simulink model "ssc_aircraft_ecs_data"  (Simulink 9.1)
settings: Solver=VariableStepAuto  StartTime=0.0  StopTime=6000  RelTol=1e-3  AbsTol=1e-3
PreLoadFcn:
  | p_init = 101.325; % kPa
  | T_init = 45; % degC
  | RH_init = 0.5;
  | O3_init = 0.05e-6;
  | 
  | R_O3 = 173.218; % J/(kg*K)
  | 
  | flow_area = 0.016; % m^2
  | 
  | D_fuselage = 4; % m
  | L_fuselage = 35; % m
undefined symbols (not defined in the file or in its folder): sigbuilder_block
libraries: fl_lib x57, nesl_utility x24, simulink x6, HVAC_lib x4
(part 2 of 2)

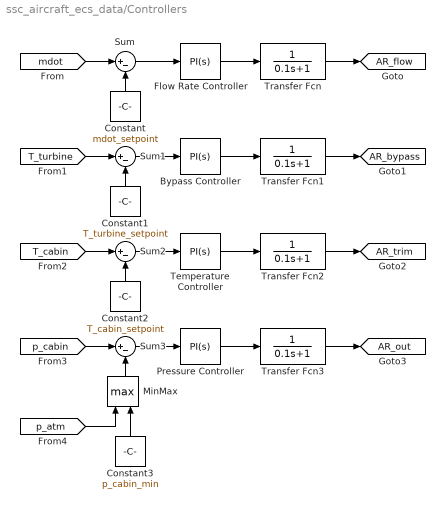
== system ssc_aircraft_ecs_data/Controllers ==
  Bypass Controller : simulink/Continuous/PID Controller  Controller=PI  TimeDomain=Continuous-time  SampleTime=-1  IntegratorMethod=Forward Euler  FilterMethod=Forward Euler  Form=Parallel  UseFilter=on  ControllerParametersSource=internal  P=-flow_area/100  I=-flow_area/100  D=0  N=100  InitialConditionSource=internal  InitialConditionForIntegrator=0  InitialConditionForFilter=0  ExternalReset=none  LimitOutput=on  UpperSaturationLimit=0.95*flow_area  LowerSaturationLimit=1e-9  LinearizeAsGain=on  AntiWindupMode=back-calculation  Kb=1  TrackingMode=off  Kt=1  PParamMin=[]  PParamMax=[]  IParamMin=[]  IParamMax=[]  DParamMin=[]  DParamMax=[]  NParamMin=[]  NParamMax=[]  KbParamMin=[]  KbParamMax=[]  KtParamMin=[]  KtParamMax=[]  POutMin=[]  POutMax=[]  IOutMin=[]  IOutMax=[]  DOutMin=[]  DOutMax=[]  NOutMin=[]  NOutMax=[]  KbOutMin=[]  KbOutMax=[]  KtOutMin=[]  KtOutMax=[]  IntegratorOutMin=[]  IntegratorOutMax=[]  FilterOutMin=[]  FilterOutMax=[]  SumOutMin=[]  SumOutMax=[]  SumI1OutMin=[]  SumI1OutMax=[]  SumI2OutMin=[]  SumI2OutMax=[]  SumI3OutMin=[]  SumI3OutMax=[]  SumDOutMin=[]  SumDOutMax=[]  SaturationOutMin=[]  SaturationOutMax=[]  IntegratorContinuousStateAttributes=''  IntegratorStateMustResolveToSignalObject=off  IntegratorRTWStateStorageClass=Auto  FilterContinuousStateAttributes=''  FilterStateMustResolveToSignalObject=off  FilterRTWStateStorageClass=Auto  DifferentiatorICPrevScaledInput=0  DifferentiatorOutMin=[]  DifferentiatorOutMax=[]  InitialConditionSetting=State (most efficient)  FilterDiffOutCoefMin=[]  FilterDiffOutCoefMax=[]  SumDenOutMin=[]  SumDenOutMax=[]  SumNumOutMin=[]  SumNumOutMax=[]  ReciprocalOutMin=[]  ReciprocalOutMax=[]  DivideOutMin=[]  DivideOutMax=[]  TunerSelectOption=Transfer Function Based (PID Tuner App)
  Constant : Constant  Value=mdot_setpoint
  Constant1 : Constant  Value=T_turbine_setpoint
  Constant2 : Constant  Value=T_cabin_setpoint
  Constant3 : Constant  Value=p_cabin_min
  Flow Rate Controller : simulink/Continuous/PID Controller  Controller=PI  TimeDomain=Continuous-time  SampleTime=-1  IntegratorMethod=Forward Euler  FilterMethod=Forward Euler  Form=Parallel  UseFilter=on  ControllerParametersSource=internal  P=-flow_area/10  I=-flow_area/10  D=0  N=100  InitialConditionSource=internal  InitialConditionForIntegrator=0  InitialConditionForFilter=0  ExternalReset=none  LimitOutput=on  UpperSaturationLimit=0.95*flow_area  LowerSaturationLimit=1e-9  LinearizeAsGain=on  AntiWindupMode=back-calculation  Kb=1  TrackingMode=off  Kt=1  PParamMin=[]  PParamMax=[]  IParamMin=[]  IParamMax=[]  DParamMin=[]  DParamMax=[]  NParamMin=[]  NParamMax=[]  KbParamMin=[]  KbParamMax=[]  KtParamMin=[]  KtParamMax=[]  POutMin=[]  POutMax=[]  IOutMin=[]  IOutMax=[]  DOutMin=[]  DOutMax=[]  NOutMin=[]  NOutMax=[]  KbOutMin=[]  KbOutMax=[]  KtOutMin=[]  KtOutMax=[]  IntegratorOutMin=[]  IntegratorOutMax=[]  FilterOutMin=[]  FilterOutMax=[]  SumOutMin=[]  SumOutMax=[]  SumI1OutMin=[]  SumI1OutMax=[]  SumI2OutMin=[]  SumI2OutMax=[]  SumI3OutMin=[]  SumI3OutMax=[]  SumDOutMin=[]  SumDOutMax=[]  SaturationOutMin=[]  SaturationOutMax=[]  IntegratorContinuousStateAttributes=''  IntegratorStateMustResolveToSignalObject=off  IntegratorRTWStateStorageClass=Auto  FilterContinuousStateAttributes=''  FilterStateMustResolveToSignalObject=off  FilterRTWStateStorageClass=Auto  DifferentiatorICPrevScaledInput=0  DifferentiatorOutMin=[]  DifferentiatorOutMax=[]  InitialConditionSetting=State (most efficient)  FilterDiffOutCoefMin=[]  FilterDiffOutCoefMax=[]  SumDenOutMin=[]  SumDenOutMax=[]  SumNumOutMin=[]  SumNumOutMax=[]  ReciprocalOutMin=[]  ReciprocalOutMax=[]  DivideOutMin=[]  DivideOutMax=[]  TunerSelectOption=Transfer Function Based (PID Tuner App)
  MinMax : MinMax  Function=max  Inputs=2
  Pressure Controller : simulink/Continuous/PID Controller  Controller=PI  TimeDomain=Continuous-time  SampleTime=-1  IntegratorMethod=Forward Euler  FilterMethod=Forward Euler  Form=Parallel  UseFilter=on  ControllerParametersSource=internal  P=flow_area/100  I=flow_area/100  D=0  N=100  InitialConditionSource=internal  InitialConditionForIntegrator=0  InitialConditionForFilter=0  ExternalReset=none  LimitOutput=on  UpperSaturationLimit=0.95*flow_area  LowerSaturationLimit=1e-9  LinearizeAsGain=on  AntiWindupMode=back-calculation  Kb=1  TrackingMode=off  Kt=1  PParamMin=[]  PParamMax=[]  IParamMin=[]  IParamMax=[]  DParamMin=[]  DParamMax=[]  NParamMin=[]  NParamMax=[]  KbParamMin=[]  KbParamMax=[]  KtParamMin=[]  KtParamMax=[]  POutMin=[]  POutMax=[]  IOutMin=[]  IOutMax=[]  DOutMin=[]  DOutMax=[]  NOutMin=[]  NOutMax=[]  KbOutMin=[]  KbOutMax=[]  KtOutMin=[]  KtOutMax=[]  IntegratorOutMin=[]  IntegratorOutMax=[]  FilterOutMin=[]  FilterOutMax=[]  SumOutMin=[]  SumOutMax=[]  SumI1OutMin=[]  SumI1OutMax=[]  SumI2OutMin=[]  SumI2OutMax=[]  SumI3OutMin=[]  SumI3OutMax=[]  SumDOutMin=[]  SumDOutMax=[]  SaturationOutMin=[]  SaturationOutMax=[]  IntegratorContinuousStateAttributes=''  IntegratorStateMustResolveToSignalObject=off  IntegratorRTWStateStorageClass=Auto  FilterContinuousStateAttributes=''  FilterStateMustResolveToSignalObject=off  FilterRTWStateStorageClass=Auto  DifferentiatorICPrevScaledInput=0  DifferentiatorOutMin=[]  DifferentiatorOutMax=[]  InitialConditionSetting=State (most efficient)  FilterDiffOutCoefMin=[]  FilterDiffOutCoefMax=[]  SumDenOutMin=[]  SumDenOutMax=[]  SumNumOutMin=[]  SumNumOutMax=[]  ReciprocalOutMin=[]  ReciprocalOutMax=[]  DivideOutMin=[]  DivideOutMax=[]  TunerSelectOption=Transfer Function Based (PID Tuner App)
  Sum{,1..3} (4 alike) : Sum  Inputs=|+-
  Temperature Controller : simulink/Continuous/PID Controller  Controller=PI  TimeDomain=Continuous-time  SampleTime=-1  IntegratorMethod=Forward Euler  FilterMethod=Forward Euler  Form=Parallel  UseFilter=on  ControllerParametersSource=internal  P=-flow_area/100  I=-flow_area/100  D=0  N=100  InitialConditionSource=internal  InitialConditionForIntegrator=0  InitialConditionForFilter=0  ExternalReset=none  LimitOutput=on  UpperSaturationLimit=0.95*flow_area  LowerSaturationLimit=1e-9  LinearizeAsGain=on  AntiWindupMode=back-calculation  Kb=1  TrackingMode=off  Kt=1  PParamMin=[]  PParamMax=[]  IParamMin=[]  IParamMax=[]  DParamMin=[]  DParamMax=[]  NParamMin=[]  NParamMax=[]  KbParamMin=[]  KbParamMax=[]  KtParamMin=[]  KtParamMax=[]  POutMin=[]  POutMax=[]  IOutMin=[]  IOutMax=[]  DOutMin=[]  DOutMax=[]  NOutMin=[]  NOutMax=[]  KbOutMin=[]  KbOutMax=[]  KtOutMin=[]  KtOutMax=[]  IntegratorOutMin=[]  IntegratorOutMax=[]  FilterOutMin=[]  FilterOutMax=[]  SumOutMin=[]  SumOutMax=[]  SumI1OutMin=[]  SumI1OutMax=[]  SumI2OutMin=[]  SumI2OutMax=[]  SumI3OutMin=[]  SumI3OutMax=[]  SumDOutMin=[]  SumDOutMax=[]  SaturationOutMin=[]  SaturationOutMax=[]  IntegratorContinuousStateAttributes=''  IntegratorStateMustResolveToSignalObject=off  IntegratorRTWStateStorageClass=Auto  FilterContinuousStateAttributes=''  FilterStateMustResolveToSignalObject=off  FilterRTWStateStorageClass=Auto  DifferentiatorICPrevScaledInput=0  DifferentiatorOutMin=[]  DifferentiatorOutMax=[]  InitialConditionSetting=State (most efficient)  FilterDiffOutCoefMin=[]  FilterDiffOutCoefMax=[]  SumDenOutMin=[]  SumDenOutMax=[]  SumNumOutMin=[]  SumNumOutMax=[]  ReciprocalOutMin=[]  ReciprocalOutMax=[]  DivideOutMin=[]  DivideOutMax=[]  TunerSelectOption=Transfer Function Based (PID Tuner App)
  Transfer Fcn{,1..3} (4 alike) : TransferFcn  Denominator=[0.1 1]
  tag scope: AR_bypass=global, AR_flow=global, AR_out=global, AR_trim=global
  wires:
  Flow Rate Controller/1 -> Transfer Fcn/1
  Sum/1 -> Flow Rate Controller/1
  Constant/1 -> Sum/2
  [mdot] -> Sum/1
  Bypass Controller/1 -> Transfer Fcn1/1
  Temperature Controller/1 -> Transfer Fcn2/1
  Pressure Controller/1 -> Transfer Fcn3/1
  Sum1/1 -> Bypass Controller/1
  [T_turbine] -> Sum1/1
  Sum2/1 -> Temperature Controller/1
  Sum3/1 -> Pressure Controller/1
  [T_cabin] -> Sum2/1
  [p_cabin] -> Sum3/1
  Constant1/1 -> Sum1/2
  Constant2/1 -> Sum2/2
  MinMax/1 -> Sum3/2
  [p_atm] -> MinMax/1
  Constant3/1 -> MinMax/2
  Transfer Fcn/1 -> [AR_flow]
  Transfer Fcn1/1 -> [AR_bypass]
  Transfer Fcn2/1 -> [AR_trim]
  Transfer Fcn3/1 -> [AR_out]

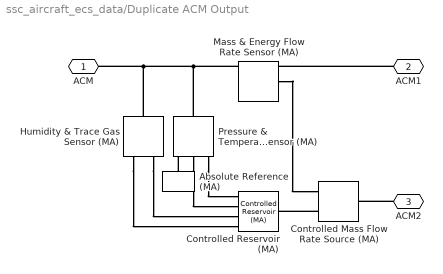
== system ssc_aircraft_ecs_data/Duplicate ACM Output ==
  Absolute Reference (MA) : fl_lib/Moist Air/Elements/Absolute Reference (MA)
      settings: SourceProductName=Simscape  SourceProductBaseCode=SS
  Controlled Mass Flow Rate Source (MA) : fl_lib/Moist Air/Sources/Controlled Mass Flow Rate Source (MA)  power_spec=foundation.enum.power_spec.none  area_A=flow_area m^2  area_B=flow_area m^2
      settings: SourceProductName=Simscape  SourceProductBaseCode=SS
  Controlled Reservoir (MA) : fl_lib/Moist Air/Elements/Controlled Reservoir (MA)  moisture_spec=foundation.enum.moisture_spec.specific_humidity  trace_gas_spec=foundation.enum.trace_gas_spec.mass_fraction  RH_ws=1  area_A=flow_area m^2  input_error_spec=foundation.enum.input_range_error.limit
      settings: SourceProductName=Simscape  SourceProductBaseCode=SS
  Humidity & Trace Gas Sensor (MA) : fl_lib/Moist Air/Sensors/Humidity & Trace Gas Sensor (MA)  moisture_spec=foundation.enum.moisture_spec.specific_humidity  trace_gas_spec=foundation.enum.trace_gas_spec.mass_fraction
      settings: SourceProductName=Simscape  SourceProductBaseCode=SS
  Mass & Energy Flow Rate Sensor (MA) : fl_lib/Moist Air/Sensors/Mass & Energy Flow Rate Sensor (MA)
      settings: SourceProductName=Simscape  SourceProductBaseCode=SS
  Pressure & Temperature Sensor (MA) : fl_lib/Moist Air/Sensors/Pressure & Temperature Sensor (MA)
      settings: SourceProductName=Simscape  SourceProductBaseCode=SS
  ACM : PMIOPort  Side=Left
  ACM1 : PMIOPort  Port=2  Side=Right
  ACM2 : PMIOPort  Port=3  Side=Right
  connections:
  ACM1/RConn1 -- Mass & Energy Flow Rate Sensor (MA)/RConn1
  Mass & Energy Flow Rate Sensor (MA)/LConn1 -- ACM/RConn1 -- Humidity & Trace Gas Sensor (MA)/LConn1 -- Pressure & Temperature Sensor (MA)/LConn1
  Controlled Mass Flow Rate Source (MA)/LConn1 -- Controlled Reservoir (MA)/LConn1
  ACM2/RConn1 -- Controlled Mass Flow Rate Source (MA)/RConn1
  Mass & Energy Flow Rate Sensor (MA)/RConn2 -- Controlled Mass Flow Rate Source (MA)/LConn2
  Humidity & Trace Gas Sensor (MA)/RConn1 -- Controlled Reservoir (MA)/RConn3
  Humidity & Trace Gas Sensor (MA)/RConn2 -- Controlled Reservoir (MA)/RConn4
  Absolute Reference (MA)/LConn1 -- Pressure & Temperature Sensor (MA)/RConn1
  Pressure & Temperature Sensor (MA)/RConn3 -- Controlled Reservoir (MA)/RConn1
  Pressure & Temperature Sensor (MA)/RConn2 -- Controlled Reservoir (MA)/RConn2

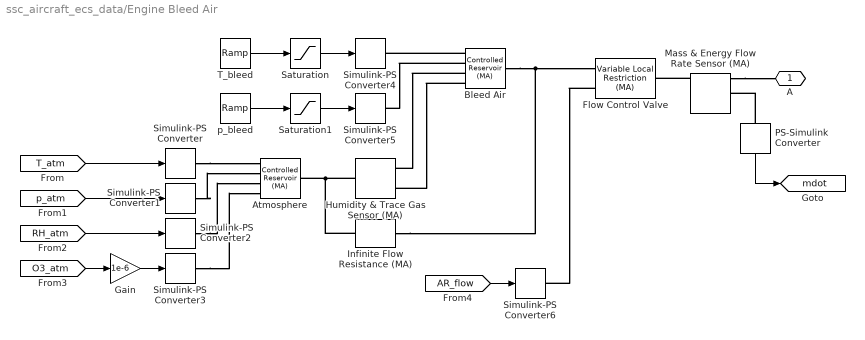
== system ssc_aircraft_ecs_data/Engine Bleed Air ==
  Atmosphere : fl_lib/Moist Air/Elements/Controlled Reservoir (MA)  moisture_spec=foundation.enum.moisture_spec.relative_humidity  trace_gas_spec=foundation.enum.trace_gas_spec.mole_fraction  RH_ws=1  area_A=flow_area m^2  input_error_spec=foundation.enum.input_range_error.warn
      settings: SourceProductName=Simscape  SourceProductBaseCode=SS
  Bleed Air : fl_lib/Moist Air/Elements/Controlled Reservoir (MA)  moisture_spec=foundation.enum.moisture_spec.specific_humidity  trace_gas_spec=foundation.enum.trace_gas_spec.mass_fraction  RH_ws=1  area_A=flow_area m^2  input_error_spec=foundation.enum.input_range_error.warn
      settings: SourceProductName=Simscape  SourceProductBaseCode=SS
  Flow Control Valve : fl_lib/Moist Air/Elements/Variable Local Restriction (MA)  min_area=1e-10 m^2  max_area=0.98*flow_area m^2  area=flow_area m^2  Cd=0.8  B_lam=0.999
      settings: SourceProductName=Simscape  SourceProductBaseCode=SS
  Gain : Gain  Gain=1e-6
  Humidity & Trace Gas Sensor (MA) : fl_lib/Moist Air/Sensors/Humidity & Trace Gas Sensor (MA)  moisture_spec=foundation.enum.moisture_spec.specific_humidity  trace_gas_spec=foundation.enum.trace_gas_spec.mass_fraction
      settings: SourceProductName=Simscape  SourceProductBaseCode=SS
  Infinite Flow Resistance (MA) : fl_lib/Moist Air/Elements/Infinite Flow Resistance (MA)  p_specify=off  p_priority=None  p=0 MPa  p_nominal_specify=off  p_nominal_unit=MPa  p_nominal_value=1  T_specify=off  T_priority=None  T=0 K  T_nominal_specify=off  T_nominal_unit=K  T_nominal_value=1  x_w_specify=off  x_w_priority=None  x_w=0  x_w_nominal_specify=off  x_w_nominal_unit=1  x_w_nominal_value=1  x_g_specify=off  x_g_priority=None  x_g=0  x_g_nominal_specify=off  x_g_nominal_unit=1  x_g_nominal_value=1
      settings: SourceProductName=Simscape  SourceProductBaseCode=SS
  Mass & Energy Flow Rate Sensor (MA) : fl_lib/Moist Air/Sensors/Mass & Energy Flow Rate Sensor (MA)
      settings: SourceProductName=Simscape  SourceProductBaseCode=SS
  PS-Simulink Converter : nesl_utility/PS-Simulink Converter  PhysicalDomain=network_engine_domain  SubClassName=ps_output  LeftPortType=input  RightPortType=output  PseudoPeriodic=off  Frequencies=[]  Unit=kg/s  AffineConversion=off
  Saturation : Saturate  UpperLimit=T_bleed  LowerLimit=-inf
  Saturation1 : Saturate  UpperLimit=p_bleed  LowerLimit=-inf
  Simulink-PS Converter : nesl_utility/Simulink-PS Converter  PhysicalDomain=network_engine_domain  SubClassName=ps_input  LeftPortType=input  RightPortType=output  PseudoPeriodic=off  Frequencies=[]  NoiseDistribution=none  NoiseParameters=[]  Unit=degC  AffineConversion=on  FilteringAndDerivatives=provide  SimscapeFilterOrder=1  InputFilterTimeConstant=0.001  UdotUserProvided=0
  Simulink-PS Converter1 : nesl_utility/Simulink-PS Converter  PhysicalDomain=network_engine_domain  SubClassName=ps_input  LeftPortType=input  RightPortType=output  PseudoPeriodic=off  Frequencies=[]  NoiseDistribution=none  NoiseParameters=[]  Unit=kPa  AffineConversion=off  FilteringAndDerivatives=provide  SimscapeFilterOrder=1  InputFilterTimeConstant=0.001  UdotUserProvided=0
  Simulink-PS Converter2 : nesl_utility/Simulink-PS Converter  PhysicalDomain=network_engine_domain  SubClassName=ps_input  LeftPortType=input  RightPortType=output  PseudoPeriodic=off  Frequencies=[]  NoiseDistribution=none  NoiseParameters=[]  Unit=1  AffineConversion=off  FilteringAndDerivatives=provide  SimscapeFilterOrder=1  InputFilterTimeConstant=0.001  UdotUserProvided=0
  Simulink-PS Converter3 : nesl_utility/Simulink-PS Converter  PhysicalDomain=network_engine_domain  SubClassName=ps_input  LeftPortType=input  RightPortType=output  PseudoPeriodic=off  Frequencies=[]  NoiseDistribution=none  NoiseParameters=[]  Unit=1  AffineConversion=off  FilteringAndDerivatives=provide  SimscapeFilterOrder=1  InputFilterTimeConstant=0.001  UdotUserProvided=0
  Simulink-PS Converter4 : nesl_utility/Simulink-PS Converter  PhysicalDomain=network_engine_domain  SubClassName=ps_input  LeftPortType=input  RightPortType=output  PseudoPeriodic=off  Frequencies=[]  NoiseDistribution=none  NoiseParameters=[]  Unit=degC  AffineConversion=on  FilteringAndDerivatives=provide  SimscapeFilterOrder=1  InputFilterTimeConstant=0.001  UdotUserProvided=0
  Simulink-PS Converter5 : nesl_utility/Simulink-PS Converter  PhysicalDomain=network_engine_domain  SubClassName=ps_input  LeftPortType=input  RightPortType=output  PseudoPeriodic=off  Frequencies=[]  NoiseDistribution=none  NoiseParameters=[]  Unit=kPa  AffineConversion=off  FilteringAndDerivatives=provide  SimscapeFilterOrder=1  InputFilterTimeConstant=0.001  UdotUserProvided=0
  Simulink-PS Converter6 : nesl_utility/Simulink-PS Converter  PhysicalDomain=network_engine_domain  SubClassName=ps_input  LeftPortType=input  RightPortType=output  PseudoPeriodic=off  Frequencies=[]  NoiseDistribution=none  NoiseParameters=[]  Unit=m^2  AffineConversion=off  FilteringAndDerivatives=provide  SimscapeFilterOrder=1  InputFilterTimeConstant=0.001  UdotUserProvided=0
  T_bleed : simulink/Sources/Ramp  slope=(T_bleed - T_init)/10  start=0  InitialOutput=T_init
  p_bleed : simulink/Sources/Ramp  slope=(p_bleed - p_init)/10  start=0  InitialOutput=p_init
  A : PMIOPort  Side=Right
  tag scope: mdot=global
  wires:
  Saturation/1 -> Simulink-PS Converter4/1
  Saturation1/1 -> Simulink-PS Converter5/1
  [T_atm] -> Simulink-PS Converter/1
  [p_atm] -> Simulink-PS Converter1/1
  [RH_atm] -> Simulink-PS Converter2/1
  [O3_atm] -> Gain/1
  [AR_flow] -> Simulink-PS Converter6/1
  PS-Simulink Converter/1 -> [mdot]
  Gain/1 -> Simulink-PS Converter3/1
  T_bleed/1 -> Saturation/1
  p_bleed/1 -> Saturation1/1
  connections:
  Flow Control Valve/LConn2 -- Simulink-PS Converter6/RConn1
  Bleed Air/LConn1 -- Infinite Flow Resistance (MA)/RConn1 -- Flow Control Valve/LConn1
  Bleed Air/RConn2 -- Simulink-PS Converter5/RConn1
  Bleed Air/RConn1 -- Simulink-PS Converter4/RConn1
  Bleed Air/RConn4 -- Humidity & Trace Gas Sensor (MA)/RConn2
  Bleed Air/RConn3 -- Humidity & Trace Gas Sensor (MA)/RConn1
  PS-Simulink Converter/LConn1 -- Mass & Energy Flow Rate Sensor (MA)/RConn2
  Humidity & Trace Gas Sensor (MA)/LConn1 -- Infinite Flow Resistance (MA)/LConn1 -- Atmosphere/LConn1
  Simulink-PS Converter/RConn1 -- Atmosphere/RConn1
  Simulink-PS Converter1/RConn1 -- Atmosphere/RConn2
  Simulink-PS Converter2/RConn1 -- Atmosphere/RConn3
  Simulink-PS Converter3/RConn1 -- Atmosphere/RConn4
  Mass & Energy Flow Rate Sensor (MA)/RConn1 -- A/RConn1
  Mass & Energy Flow Rate Sensor (MA)/LConn1 -- Flow Control Valve/RConn1

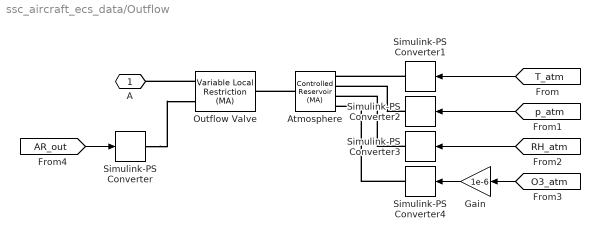
== system ssc_aircraft_ecs_data/Outflow ==
  Atmosphere : fl_lib/Moist Air/Elements/Controlled Reservoir (MA)  moisture_spec=foundation.enum.moisture_spec.relative_humidity  trace_gas_spec=foundation.enum.trace_gas_spec.mole_fraction  RH_ws=1  area_A=flow_area m^2  input_error_spec=foundation.enum.input_range_error.warn
      settings: SourceProductName=Simscape  SourceProductBaseCode=SS
  Gain : Gain  Gain=1e-6
  Outflow Valve : fl_lib/Moist Air/Elements/Variable Local Restriction (MA)  min_area=1e-10 m^2  max_area=0.98*flow_area m^2  area=flow_area m^2  Cd=0.8  B_lam=0.999
      settings: SourceProductName=Simscape  SourceProductBaseCode=SS
  Simulink-PS Converter : nesl_utility/Simulink-PS Converter  PhysicalDomain=network_engine_domain  SubClassName=ps_input  LeftPortType=input  RightPortType=output  PseudoPeriodic=off  Frequencies=[]  NoiseDistribution=none  NoiseParameters=[]  Unit=m^2  AffineConversion=off  FilteringAndDerivatives=provide  SimscapeFilterOrder=1  InputFilterTimeConstant=0.001  UdotUserProvided=0
  Simulink-PS Converter1 : nesl_utility/Simulink-PS Converter  PhysicalDomain=network_engine_domain  SubClassName=ps_input  LeftPortType=input  RightPortType=output  PseudoPeriodic=off  Frequencies=[]  NoiseDistribution=none  NoiseParameters=[]  Unit=degC  AffineConversion=on  FilteringAndDerivatives=provide  SimscapeFilterOrder=1  InputFilterTimeConstant=0.001  UdotUserProvided=0
  Simulink-PS Converter2 : nesl_utility/Simulink-PS Converter  PhysicalDomain=network_engine_domain  SubClassName=ps_input  LeftPortType=input  RightPortType=output  PseudoPeriodic=off  Frequencies=[]  NoiseDistribution=none  NoiseParameters=[]  Unit=kPa  AffineConversion=off  FilteringAndDerivatives=provide  SimscapeFilterOrder=1  InputFilterTimeConstant=0.001  UdotUserProvided=0
  Simulink-PS Converter3 : nesl_utility/Simulink-PS Converter  PhysicalDomain=network_engine_domain  SubClassName=ps_input  LeftPortType=input  RightPortType=output  PseudoPeriodic=off  Frequencies=[]  NoiseDistribution=none  NoiseParameters=[]  Unit=1  AffineConversion=off  FilteringAndDerivatives=provide  SimscapeFilterOrder=1  InputFilterTimeConstant=0.001  UdotUserProvided=0
  Simulink-PS Converter4 : nesl_utility/Simulink-PS Converter  PhysicalDomain=network_engine_domain  SubClassName=ps_input  LeftPortType=input  RightPortType=output  PseudoPeriodic=off  Frequencies=[]  NoiseDistribution=none  NoiseParameters=[]  Unit=1  AffineConversion=off  FilteringAndDerivatives=provide  SimscapeFilterOrder=1  InputFilterTimeConstant=0.001  UdotUserProvided=0
  A : PMIOPort  Side=Left
  wires:
  [T_atm] -> Simulink-PS Converter1/1
  [p_atm] -> Simulink-PS Converter2/1
  [RH_atm] -> Simulink-PS Converter3/1
  [O3_atm] -> Gain/1
  [AR_out] -> Simulink-PS Converter/1
  Gain/1 -> Simulink-PS Converter4/1
  connections:
  Atmosphere/LConn1 -- Outflow Valve/RConn1
  Outflow Valve/LConn1 -- A/RConn1
  Simulink-PS Converter2/RConn1 -- Atmosphere/RConn2
  Simulink-PS Converter1/RConn1 -- Atmosphere/RConn1
  Simulink-PS Converter3/RConn1 -- Atmosphere/RConn3
  Simulink-PS Converter4/RConn1 -- Atmosphere/RConn4
  Simulink-PS Converter/RConn1 -- Outflow Valve/LConn2

== system ssc_aircraft_ecs_data/Ram Air ==
  Constant : Constant  Value=mdot_ram
  Simulink-PS Converter : nesl_utility/Simulink-PS Converter  PhysicalDomain=network_engine_domain  SubClassName=ps_input  LeftPortType=input  RightPortType=output  PseudoPeriodic=off  Frequencies=[]  NoiseDistribution=none  NoiseParameters=[]  Unit=degC  AffineConversion=on  FilteringAndDerivatives=provide  SimscapeFilterOrder=1  InputFilterTimeConstant=0.001  UdotUserProvided=0
  Simulink-PS Converter1 : nesl_utility/Simulink-PS Converter  PhysicalDomain=network_engine_domain  SubClassName=ps_input  LeftPortType=input  RightPortType=output  PseudoPeriodic=off  Frequencies=[]  NoiseDistribution=none  NoiseParameters=[]  Unit=kg/s  AffineConversion=off  FilteringAndDerivatives=provide  SimscapeFilterOrder=1  InputFilterTimeConstant=0.001  UdotUserProvided=0
  T : PMIOPort  Side=Right
  M : PMIOPort  Port=2  Side=Right
  wires:
  [T_rec] -> Simulink-PS Converter/1
  Constant/1 -> Simulink-PS Converter1/1
  connections:
  Simulink-PS Converter/RConn1 -- T/RConn1
  Simulink-PS Converter1/RConn1 -- M/RConn1

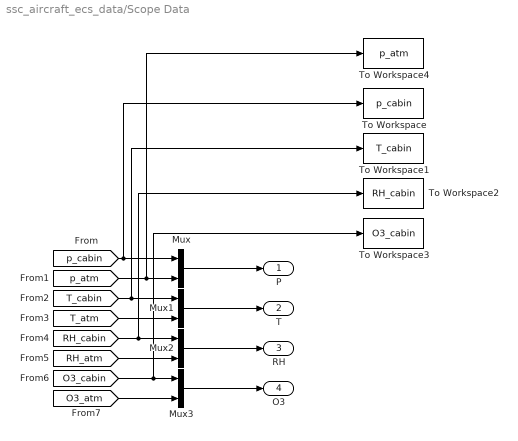
== system ssc_aircraft_ecs_data/Scope Data ==
  Mux{,1..3} (4 alike) : Mux  Inputs=2
  To Workspace : ToWorkspace  VariableName=p_cabin  SampleTime=1
  To Workspace1 : ToWorkspace  VariableName=T_cabin  SampleTime=1
  To Workspace2 : ToWorkspace  VariableName=RH_cabin  SampleTime=1
  To Workspace3 : ToWorkspace  VariableName=O3_cabin  SampleTime=1
  To Workspace4 : ToWorkspace  VariableName=p_atm  SampleTime=1
  P : Outport
  T : Outport  Port=2
  RH : Outport  Port=3
  O3 : Outport  Port=4
  wires:
  [p_cabin] -> To Workspace/1, Mux/1
  [T_atm] -> Mux1/2
  [p_atm] -> To Workspace4/1, Mux/2
  [RH_atm] -> Mux2/2
  [T_cabin] -> To Workspace1/1, Mux1/1
  [O3_cabin] -> To Workspace3/1, Mux3/1
  [RH_cabin] -> To Workspace2/1, Mux2/1
  [O3_atm] -> Mux3/2
  Mux2/1 -> RH/1
  Mux/1 -> P/1
  Mux1/1 -> T/1
  Mux3/1 -> O3/1

== system ssc_aircraft_ecs_data/T,s 1 ==
  Thermodynamic Properties Sensor (MA) : fl_lib/Moist Air/Sensors/Thermodynamic Properties Sensor (MA)
      settings: SourceProductName=Simscape  SourceProductBaseCode=SS
  A : PMIOPort  Side=Left
  connections:
  Thermodynamic Properties Sensor (MA)/LConn1 -- A/RConn1

== system ssc_aircraft_ecs_data/T,s 2 ==
  Thermodynamic Properties Sensor (MA) : fl_lib/Moist Air/Sensors/Thermodynamic Properties Sensor (MA)
      settings: SourceProductName=Simscape  SourceProductBaseCode=SS
  A : PMIOPort  Side=Left
  connections:
  Thermodynamic Properties Sensor (MA)/LConn1 -- A/RConn1

== system ssc_aircraft_ecs_data/T,s 3 ==
  Thermodynamic Properties Sensor (MA) : fl_lib/Moist Air/Sensors/Thermodynamic Properties Sensor (MA)
      settings: SourceProductName=Simscape  SourceProductBaseCode=SS
  A : PMIOPort  Side=Left
  connections:
  Thermodynamic Properties Sensor (MA)/LConn1 -- A/RConn1

== system ssc_aircraft_ecs_data/T,s 4 ==
  Thermodynamic Properties Sensor (MA) : fl_lib/Moist Air/Sensors/Thermodynamic Properties Sensor (MA)
      settings: SourceProductName=Simscape  SourceProductBaseCode=SS
  A : PMIOPort  Side=Left
  connections:
  Thermodynamic Properties Sensor (MA)/LConn1 -- A/RConn1

== system ssc_aircraft_ecs_data/T,s 5 ==
  Absolute Reference (MA) : fl_lib/Moist Air/Elements/Absolute Reference (MA)
      settings: SourceProductName=Simscape  SourceProductBaseCode=SS
  PS-Simulink Converter : nesl_utility/PS-Simulink Converter  PhysicalDomain=network_engine_domain  SubClassName=ps_output  LeftPortType=input  RightPortType=output  PseudoPeriodic=off  Frequencies=[]  Unit=degC  AffineConversion=on
  Pressure & Temperature Sensor (MA) : fl_lib/Moist Air/Sensors/Pressure & Temperature Sensor (MA)
      settings: SourceProductName=Simscape  SourceProductBaseCode=SS
  Thermodynamic Properties Sensor (MA) : fl_lib/Moist Air/Sensors/Thermodynamic Properties Sensor (MA)
      settings: SourceProductName=Simscape  SourceProductBaseCode=SS
  A : PMIOPort  Side=Left
  tag scope: T_turbine=global
  wires:
  PS-Simulink Converter/1 -> [T_turbine]
  connections:
  Thermodynamic Properties Sensor (MA)/LConn1 -- A/RConn1 -- Pressure & Temperature Sensor (MA)/LConn1
  Pressure & Temperature Sensor (MA)/RConn3 -- PS-Simulink Converter/LConn1
  Absolute Reference (MA)/LConn1 -- Pressure & Temperature Sensor (MA)/RConn1

== system ssc_aircraft_ecs_data/T,s 6 ==
  Thermodynamic Properties Sensor (MA) : fl_lib/Moist Air/Sensors/Thermodynamic Properties Sensor (MA)
      settings: SourceProductName=Simscape  SourceProductBaseCode=SS
  A : PMIOPort  Side=Left
  connections:
  Thermodynamic Properties Sensor (MA)/LConn1 -- A/RConn1

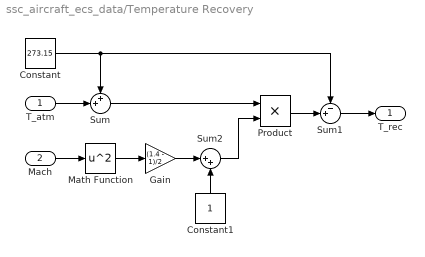
== system ssc_aircraft_ecs_data/Temperature Recovery ==
  T_atm : Inport
  Mach : Inport  Port=2
  Constant : Constant  Value=273.15
  Constant1 : Constant
  Gain : Gain  Gain=(1.4 - 1)/2
  Math Function : Math  Operator=square  SaturateOnIntegerOverflow=on
  Product : Product
  Sum : Sum  Inputs=++|
  Sum1 : Sum  Inputs=-+|
  Sum2 : Sum  Inputs=|++
  T_rec : Outport
  wires:
  T_atm/1 -> Sum/2
  Sum1/1 -> T_rec/1
  Constant/1 -> Sum1/1, Sum/1
  Mach/1 -> Math Function/1
  Math Function/1 -> Gain/1
  Gain/1 -> Sum2/1
  Constant1/1 -> Sum2/2
  Product/1 -> Sum1/2
  Sum2/1 -> Product/2
  Sum/1 -> Product/1

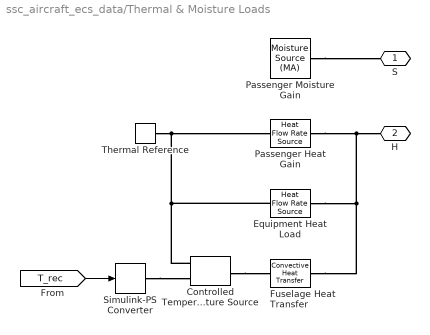
== system ssc_aircraft_ecs_data/Thermal & Moisture Loads ==
  Controlled Temperature Source : fl_lib/Thermal/Thermal Sources/Controlled Temperature Source
      settings: SourceProductName=Simscape
  Equipment Heat Load : fl_lib/Thermal/Thermal Sources/Heat Flow Rate Source  heat_flow=Q_equipment W
      settings: SourceProductName=Simscape  SourceProductBaseCode=SS
  Fuselage Heat Transfer : fl_lib/Thermal/Thermal Elements/Convective Heat Transfer  area=pi * D_fuselage * L_fuselage m^2  heat_tr_coeff=hc_fuselage W/(m^2 * K)  T_specify=off  T_priority=None  T=0 K  T_nominal_specify=off  T_nominal_unit=K  T_nominal_value=1  Q_specify=off  Q_priority=None  Q=0 W  Q_nominal_specify=off  Q_nominal_unit=W  Q_nominal_value=1
  Passenger Heat Gain : fl_lib/Thermal/Thermal Sources/Heat Flow Rate Source  heat_flow=Q_passenger * N_passenger W
      settings: SourceProductName=Simscape  SourceProductBaseCode=SS
  Passenger Moisture Gain : fl_lib/Moist Air/Sources/Moisture & Trace Gas Sources/Moisture Source (MA)  moisture_source_spec=foundation.enum.moisture_source_spec.vapor  moisture_mass_flow=W_passenger * N_passenger g/s  temperature_spec=2  moisture_temperature=T_passenger degC
      settings: SourceProductName=Simscape  SourceProductBaseCode=SS
  Simulink-PS Converter : nesl_utility/Simulink-PS Converter  PhysicalDomain=network_engine_domain  SubClassName=ps_input  LeftPortType=input  RightPortType=output  PseudoPeriodic=off  Frequencies=[]  NoiseDistribution=none  NoiseParameters=[]  Unit=degC  AffineConversion=on  FilteringAndDerivatives=provide  SimscapeFilterOrder=1  InputFilterTimeConstant=0.001  UdotUserProvided=0
  Thermal Reference : fl_lib/Thermal/Thermal Elements/Thermal Reference
  S : PMIOPort  Side=Right
  H : PMIOPort  Port=2  Side=Right
  wires:
  [T_rec] -> Simulink-PS Converter/1
  connections:
  Passenger Moisture Gain/LConn1 -- S/RConn1
  Passenger Heat Gain/LConn1 -- Equipment Heat Load/LConn1 -- Fuselage Heat Transfer/RConn1 -- H/RConn1
  Controlled Temperature Source/LConn1 -- Fuselage Heat Transfer/LConn1
  Thermal Reference/LConn1 -- Equipment Heat Load/RConn1 -- Controlled Temperature Source/RConn2 -- Passenger Heat Gain/RConn1
  Simulink-PS Converter/RConn1 -- Controlled Temperature Source/RConn1

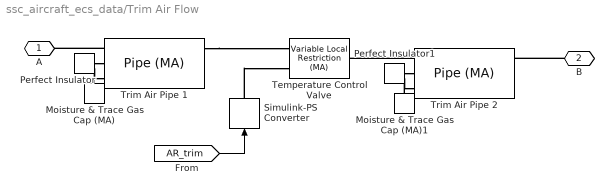
== system ssc_aircraft_ecs_data/Trim Air Flow ==
  Moisture & Trace Gas Cap (MA) : fl_lib/Moist Air/Sources/Moisture & Trace Gas Sources/Moisture & Trace Gas Cap (MA)
      settings: SourceProductName=Simscape  SourceProductBaseCode=SS
  Moisture & Trace Gas Cap (MA)1 : fl_lib/Moist Air/Sources/Moisture & Trace Gas Sources/Moisture & Trace Gas Cap (MA)
      settings: SourceProductName=Simscape  SourceProductBaseCode=SS
  Perfect Insulator : fl_lib/Thermal/Thermal Elements/Perfect Insulator  T_specify=off  T_priority=None  T=0 K  T_nominal_specify=off  T_nominal_unit=K  T_nominal_value=1
      settings: SourceProductName=Simscape
  Perfect Insulator1 : fl_lib/Thermal/Thermal Elements/Perfect Insulator  T_specify=off  T_priority=None  T=0 K  T_nominal_specify=off  T_nominal_unit=K  T_nominal_value=1
      settings: SourceProductName=Simscape
  Simulink-PS Converter : nesl_utility/Simulink-PS Converter  PhysicalDomain=network_engine_domain  SubClassName=ps_input  LeftPortType=input  RightPortType=output  PseudoPeriodic=off  Frequencies=[]  NoiseDistribution=none  NoiseParameters=[]  Unit=m^2  AffineConversion=off  FilteringAndDerivatives=provide  SimscapeFilterOrder=1  InputFilterTimeConstant=0.001  UdotUserProvided=0
  Temperature Control Valve : fl_lib/Moist Air/Elements/Variable Local Restriction (MA)  min_area=1e-10 m^2  max_area=0.98*flow_area m^2  area=flow_area m^2  Cd=0.8  B_lam=0.999
      settings: SourceProductName=Simscape  SourceProductBaseCode=SS
  Trim Air Pipe 1 : fl_lib/Moist Air/Elements/Pipe (MA)  length=1 m  area=flow_area m^2  Dh=sqrt(flow_area*4/pi) m  length_add=0.1 m  roughness=15e-6 m  Re_lam=2000  Re_tur=4000  shape_factor=64  Nu_lam=3.66  RH_ws=1  time_constant=1e-3 s  p_I_specify=on  p_I_priority=High  p_I=p_init kPa  p_I_nominal_specify=off  p_I_nominal_unit=MPa  p_I_nominal_value=1  T_I_specify=on  T_I_priority=High  T_I=T_init degC  T_I_nominal_specify=off  T_I_nominal_unit=K  T_I_nominal_value=1  RH_I_specify=on  RH_I_priority=High  RH_I=RH_init  RH_I_nominal_specify=off  RH_I_nominal_unit=1  RH_I_nominal_value=1  x_w_I_specify=off  x_w_I_priority=None  x_w_I=0  x_w_I_nominal_specify=off  x_w_I_nominal_unit=1  x_w_I_nominal_value=1  y_w_I_specify=off  y_w_I_priority=None  y_w_I=0  y_w_I_nominal_specify=off  y_w_I_nominal_unit=1  y_w_I_nominal_value=1  HR_I_specify=off  HR_I_priority=None  HR_I=0  HR_I_nominal_specify=off  HR_I_nominal_unit=1  HR_I_nominal_value=1  x_g_I_specify=on  x_g_I_priority=None  x_g_I=0  x_g_I_nominal_specify=off  x_g_I_nominal_unit=1  x_g_I_nominal_value=1  y_g_I_specify=on  y_g_I_priority=High  y_g_I=O3_init  y_g_I_nominal_specify=off  y_g_I_nominal_unit=1  y_g_I_nominal_value=1  t_specify=off  t_priority=High  t=0 s  t_nominal_specify=off  t_nominal_unit=s  t_nominal_value=1
      settings: SourceProductName=Simscape  SourceProductBaseCode=SS
  Trim Air Pipe 2 : fl_lib/Moist Air/Elements/Pipe (MA)  length=1 m  area=flow_area m^2  Dh=sqrt(flow_area*4/pi) m  length_add=0.1 m  roughness=15e-6 m  Re_lam=2000  Re_tur=4000  shape_factor=64  Nu_lam=3.66  RH_ws=1  time_constant=1e-3 s  p_I_specify=on  p_I_priority=High  p_I=p_init kPa  p_I_nominal_specify=off  p_I_nominal_unit=MPa  p_I_nominal_value=1  T_I_specify=on  T_I_priority=High  T_I=T_init degC  T_I_nominal_specify=off  T_I_nominal_unit=K  T_I_nominal_value=1  RH_I_specify=on  RH_I_priority=High  RH_I=RH_init  RH_I_nominal_specify=off  RH_I_nominal_unit=1  RH_I_nominal_value=1  x_w_I_specify=off  x_w_I_priority=None  x_w_I=0  x_w_I_nominal_specify=off  x_w_I_nominal_unit=1  x_w_I_nominal_value=1  y_w_I_specify=off  y_w_I_priority=None  y_w_I=0  y_w_I_nominal_specify=off  y_w_I_nominal_unit=1  y_w_I_nominal_value=1  HR_I_specify=off  HR_I_priority=None  HR_I=0  HR_I_nominal_specify=off  HR_I_nominal_unit=1  HR_I_nominal_value=1  x_g_I_specify=on  x_g_I_priority=None  x_g_I=0  x_g_I_nominal_specify=off  x_g_I_nominal_unit=1  x_g_I_nominal_value=1  y_g_I_specify=on  y_g_I_priority=High  y_g_I=O3_init  y_g_I_nominal_specify=off  y_g_I_nominal_unit=1  y_g_I_nominal_value=1  t_specify=off  t_priority=High  t=0 s  t_nominal_specify=off  t_nominal_unit=s  t_nominal_value=1
      settings: SourceProductName=Simscape  SourceProductBaseCode=SS
  A : PMIOPort  Side=Left
  B : PMIOPort  Port=2  Side=Right
  wires:
  [AR_trim] -> Simulink-PS Converter/1
  connections:
  Simulink-PS Converter/RConn1 -- Temperature Control Valve/LConn2
  B/RConn1 -- Trim Air Pipe 2/RConn1
  Trim Air Pipe 2/LConn1 -- Temperature Control Valve/RConn1
  Moisture & Trace Gas Cap (MA)1/LConn1 -- Trim Air Pipe 2/LConn3
  Perfect Insulator1/LConn1 -- Trim Air Pipe 2/LConn2
  Perfect Insulator/LConn1 -- Trim Air Pipe 1/LConn2
  Moisture & Trace Gas Cap (MA)/LConn1 -- Trim Air Pipe 1/LConn3
  Trim Air Pipe 1/RConn1 -- Temperature Control Valve/LConn1
  Trim Air Pipe 1/LConn1 -- A/RConn1
